simulink library "BLE_Library"  (R2017b)
settings: Solver=VariableStepAuto  StartTime=0.0  StopTime=10.0  RelTol=1e-3
values from neighbouring files (symbols this model uses):
  D = D/ScaleCoefficient    [BLE_PostLoad.m]    (also in new_BLE_model.m = zeros(N_BLE,N_BLE+1))
undefined symbols (not defined in the file or in its folder): ADV_IND_AccA, ADV_IND_id, BT_Hop_Separation, BT_Samples_Per_Symbol, CONNECT_IND_id, CONNECT_IND_length, F3B672D172DF, F506B10B1B3E, Header, LL_DATA_EMPTY_length, LL_DATA_id, magnitude, Payload, Preamble, Slot_Ts, T_IFS
libraries: BLE_Library x56, simulink x39, commutil2 x29, dspindex x17, commdigbbndfm2 x5, dspsigops x2, commrandsrc3 x2, dspstat3 x2, dspsrcs4 x1, dsparch4 x1, commdigbbndcpm2 x1
(part 4 of 5)

== system BLE_Library/Demodulation, De-whitening, CRC check, PDU/De-whitening, CRC check, Data fields/De-whitening/Subsystem ==
  ChIdx : Inport
  Enable : EnablePort  StatesWhenEnabling=reset
  Initial LFSR generation : MATLAB Function  TreatAsAtomicUnit=on
  LFSR : Outport
  wires:
  ChIdx/1 -> Initial LFSR generation/1(ChIdx)
  Initial LFSR generation/1(LFSR) -> LFSR/1

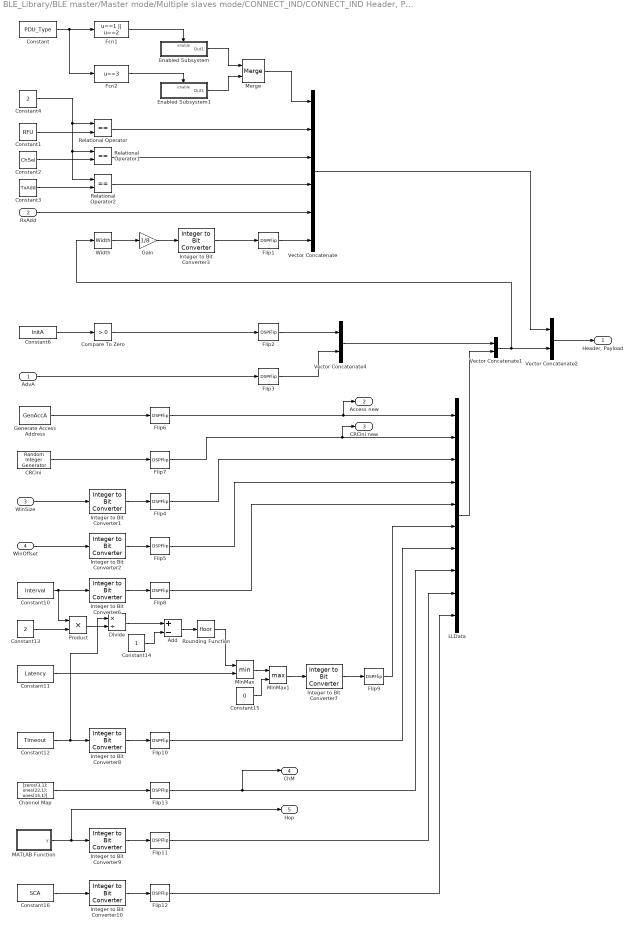
== system BLE_Library/BLE master/Master mode/Multiple slaves mode/CONNECT_IND/CONNECT_IND Header, Payload ==
  AdvA : Inport
  RxAdd : Inport  Port=2
  WinSize : Inport  Port=3
  WinOffset : Inport  Port=4
  Add : Sum  Inputs=+-
  CRCini : commrandsrc3/Random Integer Generator  SetSize=2  SeedSource=Auto  Seed=0  SampleTime=Slot_Ts/24  SamplesPerFrame=24  OutputDataType=boolean  SimulateUsing=Interpreted execution
  Channel Map : Constant  Value=[zeros(3,1); ones(22,1); ones(15,1)]  OutDataTypeStr=boolean  SampleTime=Slot_Ts
  Compare To Zero : simulink/Logic and Bit Operations/Compare To Zero  relop=>  OutDataTypeStr=boolean
  Constant : Constant  Value=PDU_Type  SampleTime=Slot_Ts
  Constant1 : Constant  Value=RFU  SampleTime=Slot_Ts
  Constant10 : Constant  Value=Interval  SampleTime=Slot_Ts
  Constant11 : Constant  Value=Latency  SampleTime=Slot_Ts
  Constant12 : Constant  Value=Timeout  SampleTime=Slot_Ts
  Constant13 : Constant  Value=2  SampleTime=Slot_Ts
  Constant14 : Constant  SampleTime=Slot_Ts
  Constant15 : Constant  Value=0  SampleTime=Slot_Ts
  Constant16 : Constant  Value=SCA  SampleTime=Slot_Ts
  Constant2 : Constant  Value=ChSel  SampleTime=Slot_Ts
  Constant3 : Constant  Value=TxAdd  SampleTime=Slot_Ts
  Constant4 : Constant  Value=2  SampleTime=Slot_Ts
  Constant6 : Constant  Value=InitA  VectorParams1D=off  OutDataTypeStr=double  SampleTime=Slot_Ts
  Divide : Product  Inputs=*/
  Enabled Subsystem : Subsystem  TreatAsAtomicUnit=on
  Enabled Subsystem1 : Subsystem  TreatAsAtomicUnit=on
  Fcn1 : Fcn  Expr=u==1 || u==2
  Fcn2 : Fcn  Expr=u==3
  Flip{1..13} (13 alike) : DSPFlip
  Gain : Gain  Gain=1/8
  Generate Access Address : M-S-Function  Priority=2  FunctionName=GenAccA  Parameters=Slot_Ts
  Integer to Bit Converter1 : commutil2/Integer to Bit Converter  nbits=8  signedInputValues=Unsigned  bitOrder=MSB first  outDtype=boolean
  Integer to Bit Converter10 : commutil2/Integer to Bit Converter  nbits=3  signedInputValues=Unsigned  bitOrder=MSB first  outDtype=boolean
  Integer to Bit Converter{2,6..8} (4 alike) : commutil2/Integer to Bit Converter  nbits=16  signedInputValues=Unsigned  bitOrder=MSB first  outDtype=boolean
  Integer to Bit Converter3 : commutil2/Integer to Bit Converter  nbits=8  signedInputValues=Unsigned  bitOrder=MSB first  outDtype=boolean
  Integer to Bit Converter9 : commutil2/Integer to Bit Converter  nbits=5  signedInputValues=Unsigned  bitOrder=MSB first  outDtype=boolean
  LLData : Concatenate  NumInputs=10
  MATLAB Function : MATLAB Function  TreatAsAtomicUnit=on
  Merge : Merge
  MinMax : MinMax  Inputs=2
  MinMax1 : MinMax  Function=max  Inputs=2
  Product : Product
  Relational Operator : RelationalOperator  Operator===  OutDataTypeStr=boolean  RndMeth=Simplest
  Relational Operator1 : RelationalOperator  Operator===  OutDataTypeStr=boolean  RndMeth=Simplest
  Relational Operator2 : RelationalOperator  Operator===  OutDataTypeStr=boolean  RndMeth=Simplest
  Rounding Function : Rounding
  Vector Concatenate : Concatenate  NumInputs=6
  Vector Concatenate1 : Concatenate
  Vector Concatenate2 : Concatenate
  Vector Concatenate4 : Concatenate
  Width : Width
  "Header, Payload" : Outport
  Access new : Outport  Port=2
  CRCini new : Outport  Port=3
  ChM : Outport  Port=4
  Hop : Outport  Port=5
  wires:
  WinOffset/1 -> Integer to Bit Converter2/1
  WinSize/1 -> Integer to Bit Converter1/1
  MATLAB Function/1(y) -> Integer to Bit Converter9/1, Hop/1
  Channel Map/1 -> Flip13/1
  Flip13/1 -> LLData/8, ChM/1
  Constant14/1 -> Add/2
  Constant11/1 -> MinMax/2
  Constant6/1 -> Compare To Zero/1
  Integer to Bit Converter2/1 -> Flip5/1
  Flip5/1 -> LLData/4
  Fcn1/1 -> Enabled Subsystem/Enable
  Product/1 -> Divide/2
  Merge/1 -> Vector Concatenate/1
  Vector Concatenate/1 -> Vector Concatenate2/1
  Integer to Bit Converter7/1 -> Flip9/1
  Constant/1 -> Fcn1/1, Fcn2/1
  Flip7/1 -> CRCini new/1, LLData/2
  Vector Concatenate2/1 -> "Header, Payload"/1
  Constant1/1 -> Relational Operator/2
  Gain/1 -> Integer to Bit Converter3/1
  Constant4/1 -> Relational Operator2/1, Relational Operator1/1, Relational Operator/1
  CRCini/1 -> Flip7/1
  Integer to Bit Converter8/1 -> Flip10/1
  Integer to Bit Converter9/1 -> Flip11/1
  Flip6/1 -> Access new/1, LLData/1
  Integer to Bit Converter1/1 -> Flip4/1
  MinMax1/1 -> Integer to Bit Converter7/1
  AdvA/1 -> Flip3/1
  Constant13/1 -> Product/2
  Enabled Subsystem/1(Out1) -> Merge/1
  Integer to Bit Converter10/1 -> Flip12/1
  Constant10/1 -> Product/1, Integer to Bit Converter6/1
  Constant3/1 -> Relational Operator2/2
  Divide/1 -> Add/1
  Flip12/1 -> LLData/10
  MinMax/1 -> MinMax1/1
  Enabled Subsystem1/1(Out1) -> Merge/2
  Integer to Bit Converter6/1 -> Flip8/1
  Flip1/1 -> Vector Concatenate/6
  Fcn2/1 -> Enabled Subsystem1/Enable
  Add/1 -> Rounding Function/1
  Relational Operator/1 -> Vector Concatenate/2
  Width/1 -> Gain/1
  Flip4/1 -> LLData/3
  Vector Concatenate4/1 -> Vector Concatenate1/1
  Constant12/1 -> Divide/1, Integer to Bit Converter8/1
  Flip8/1 -> LLData/5
  Vector Concatenate1/1 -> Width/1, Vector Concatenate2/2
  Relational Operator2/1 -> Vector Concatenate/4
  Flip11/1 -> LLData/9
  Flip9/1 -> LLData/6
  Constant16/1 -> Integer to Bit Converter10/1
  Flip10/1 -> LLData/7
  Constant2/1 -> Relational Operator1/2
  Constant15/1 -> MinMax1/2
  Flip3/1 -> Vector Concatenate4/2
  LLData/1 -> Vector Concatenate1/2
  Flip2/1 -> Vector Concatenate4/1
  Integer to Bit Converter3/1 -> Flip1/1
  Relational Operator1/1 -> Vector Concatenate/3
  RxAdd/1 -> Vector Concatenate/5
  Generate Access Address/1 -> Flip6/1
  Compare To Zero/1 -> Flip2/1
  Rounding Function/1 -> MinMax/1

== system BLE_Library/BLE master/Master mode/Multiple slaves mode/CONNECT_IND/Subsystem4 ==
  AdvAccAdr : Constant  Value=ADV_IND_AccA  VectorParams1D=off  SampleTime=Slot_Ts
  AdvPreamble : Constant  Value=[0 1 0 1 0 1 0 1]'  VectorParams1D=off  OutDataTypeStr=boolean  SampleTime=Slot_Ts  FramePeriod=Slot_Ts
  "Concatenate Adv Preamble, Access address" : Concatenate  Mode=Multidimensional array
  Flip1 : DSPFlip
  Out1 : Outport
  wires:
  Flip1/1 -> "Concatenate Adv Preamble, Access address"/2
  AdvPreamble/1 -> "Concatenate Adv Preamble, Access address"/1
  "Concatenate Adv Preamble, Access address"/1 -> Out1/1
  AdvAccAdr/1 -> Flip1/1

== system BLE_Library/BLE master/Master mode/Multiple slaves mode/Subsystem/If Action Subsystem ==
  Header : Inport
  PDU : Inport  Port=2
  Action Port : ActionPort
  Constant : Constant  OutDataTypeStr=boolean  SampleTime=Slot_Ts
  Multiport Selector : dspindex/Multiport Selector  rowsOrCols=Rows  idxCellArray={1:48}  idxErrMode=Clip Index
  Multiport Selector1 : dspindex/Multiport Selector  rowsOrCols=Rows  idxCellArray={10}  idxErrMode=Clip Index
  TxAdd : Outport
  AdvA : Outport  Port=2
  ADV OK : Outport  Port=3
  wires:
  Constant/1 -> ADV OK/1
  Header/1 -> Multiport Selector1/1
  Multiport Selector1/1 -> TxAdd/1
  PDU/1 -> Multiport Selector/1
  Multiport Selector/1 -> AdvA/1

== system BLE_Library/BLE master/Master mode/Multiple slaves mode/Subsystem/If Action Subsystem1 ==
  Header : Inport
  PDU : Inport  Port=2
  Action Port : ActionPort
  Compare To Constant : simulink/Logic and Bit Operations/Compare To Constant  relop===  const=48  OutDataTypeStr=boolean
  Compare To Constant1 : simulink/Logic and Bit Operations/Compare To Constant  relop===  const=2  OutDataTypeStr=boolean
  Constant1 : Constant  Value=TxAdd  VectorParams1D=off  OutDataTypeStr=double  SampleTime=Slot_Ts
  Constant2 : Constant  Value=InitA  VectorParams1D=off  OutDataTypeStr=double  SampleTime=Slot_Ts
  Logical Operator : Logic  AllPortsSameDT=off  OutDataTypeStr=boolean
  Multiport Selector : dspindex/Multiport Selector  rowsOrCols=Rows  idxCellArray={1:48, 49:96}  idxErrMode=Clip Index
  Multiport Selector2 : dspindex/Multiport Selector  rowsOrCols=Rows  idxCellArray={9, 10}  idxErrMode=Clip Index
  Relational Operator1 : RelationalOperator  Operator===  OutDataTypeStr=boolean  RndMeth=Simplest
  Relational Operator2 : RelationalOperator  Operator===  OutDataTypeStr=boolean  RndMeth=Simplest
  Sum of Elements1 : Sum  Inputs=+
  ADV OK : Outport
  AdvA : Outport  Port=2
  TxAdd : Outport  Port=3
  wires:
  Compare To Constant1/1 -> Relational Operator2/1
  Logical Operator/1 -> ADV OK/1
  Constant2/1 -> Relational Operator1/2
  Constant1/1 -> Compare To Constant1/1
  Multiport Selector2/1 -> Relational Operator2/2  "RxAdd"
  Multiport Selector/1 -> Relational Operator1/1  "TargA"
  Sum of Elements1/1 -> Compare To Constant/1
  Relational Operator2/1 -> Logical Operator/1
  Compare To Constant/1 -> Logical Operator/2
  Relational Operator1/1 -> Sum of Elements1/1
  Multiport Selector2/2 -> TxAdd/1
  Header/1 -> Multiport Selector2/1
  Multiport Selector/2 -> AdvA/1
  PDU/1 -> Multiport Selector/1

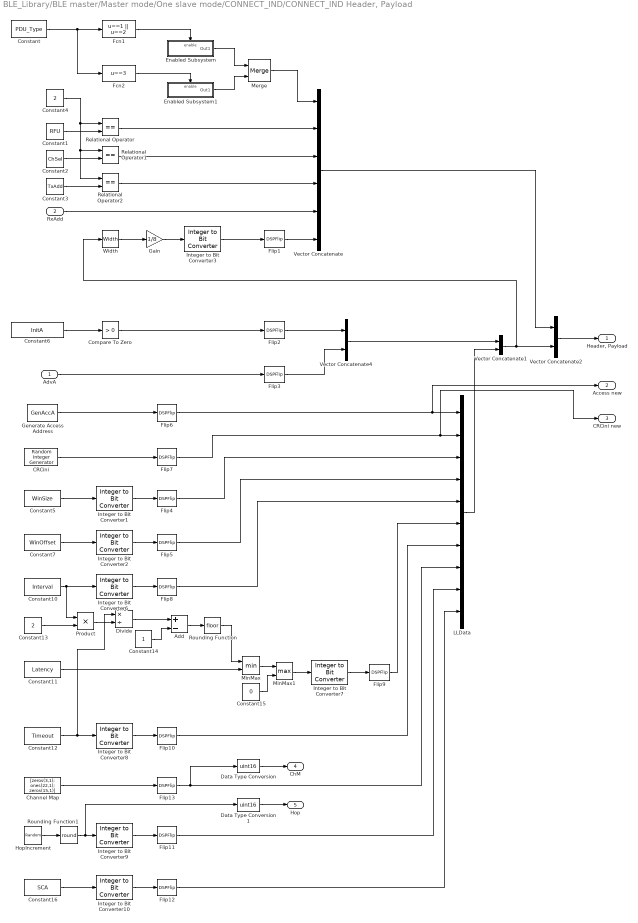
== system BLE_Library/BLE master/Master mode/One slave mode/CONNECT_IND/CONNECT_IND Header, Payload ==
  AdvA : Inport
  RxAdd : Inport  Port=2
  Add : Sum  Inputs=+-
  CRCini : commrandsrc3/Random Integer Generator  SetSize=2  SeedSource=Parameter  Seed=nD  SampleTime=Slot_Ts/24  SamplesPerFrame=24  OutputDataType=boolean  SimulateUsing=Interpreted execution
  Channel Map : Constant  Value=[zeros(3,1); ones(22,1); zeros(15,1)]  OutDataTypeStr=boolean  SampleTime=Slot_Ts
  Compare To Zero : simulink/Logic and Bit Operations/Compare To Zero  relop=>  OutDataTypeStr=boolean
  Constant : Constant  Value=PDU_Type  SampleTime=Slot_Ts
  Constant1 : Constant  Value=RFU  SampleTime=Slot_Ts
  Constant10 : Constant  Value=Interval  SampleTime=Slot_Ts
  Constant11 : Constant  Value=Latency  SampleTime=Slot_Ts
  Constant12 : Constant  Value=Timeout  SampleTime=Slot_Ts
  Constant13 : Constant  Value=2  SampleTime=Slot_Ts
  Constant14 : Constant  SampleTime=Slot_Ts
  Constant15 : Constant  Value=0  SampleTime=Slot_Ts
  Constant16 : Constant  Value=SCA  SampleTime=Slot_Ts
  Constant2 : Constant  Value=ChSel  SampleTime=Slot_Ts
  Constant3 : Constant  Value=TxAdd  SampleTime=Slot_Ts
  Constant4 : Constant  Value=2  SampleTime=Slot_Ts
  Constant5 : Constant  Value=WinSize  SampleTime=Slot_Ts
  Constant6 : Constant  Value=InitA  VectorParams1D=off  OutDataTypeStr=double  SampleTime=Slot_Ts
  Constant7 : Constant  Value=WinOffset  SampleTime=Slot_Ts
  Data Type Conversion : DataTypeConversion  OutDataTypeStr=uint16
  Data Type Conversion1 : DataTypeConversion  OutDataTypeStr=uint16
  Divide : Product  Inputs=*/
  Enabled Subsystem : Subsystem  TreatAsAtomicUnit=on
  Enabled Subsystem1 : Subsystem  TreatAsAtomicUnit=on
  Fcn1 : Fcn  Expr=u==1 || u==2
  Fcn2 : Fcn  Expr=u==3
  Flip{1..13} (13 alike) : DSPFlip
  Gain : Gain  Gain=1/8
  Generate Access Address : M-S-Function  Priority=2  FunctionName=GenAccA  Parameters=Slot_Ts
  HopIncrement : UniformRandomNumber  Minimum=5  Maximum=16  Seed=nD  SampleTime=Slot_Ts
  Integer to Bit Converter1 : commutil2/Integer to Bit Converter  nbits=8  signedInputValues=Unsigned  bitOrder=MSB first  outDtype=boolean
  Integer to Bit Converter10 : commutil2/Integer to Bit Converter  nbits=3  signedInputValues=Unsigned  bitOrder=MSB first  outDtype=boolean
  Integer to Bit Converter{2,6..8} (4 alike) : commutil2/Integer to Bit Converter  nbits=16  signedInputValues=Unsigned  bitOrder=MSB first  outDtype=boolean
  Integer to Bit Converter3 : commutil2/Integer to Bit Converter  nbits=8  signedInputValues=Unsigned  bitOrder=MSB first  outDtype=boolean
  Integer to Bit Converter9 : commutil2/Integer to Bit Converter  nbits=5  signedInputValues=Unsigned  bitOrder=MSB first  outDtype=boolean
  LLData : Concatenate  NumInputs=10
  Merge : Merge
  MinMax : MinMax  Inputs=2
  MinMax1 : MinMax  Function=max  Inputs=2
  Product : Product
  Relational Operator : RelationalOperator  Operator===  OutDataTypeStr=boolean  RndMeth=Simplest
  Relational Operator1 : RelationalOperator  Operator===  OutDataTypeStr=boolean  RndMeth=Simplest
  Relational Operator2 : RelationalOperator  Operator===  OutDataTypeStr=boolean  RndMeth=Simplest
  Rounding Function : Rounding
  Rounding Function1 : Rounding  Operator=round
  Vector Concatenate : Concatenate  NumInputs=6
  Vector Concatenate1 : Concatenate
  Vector Concatenate2 : Concatenate
  Vector Concatenate4 : Concatenate
  Width : Width
  "Header, Payload" : Outport
  Access new : Outport  Port=2
  CRCini new : Outport  Port=3
  ChM : Outport  Port=4
  Hop : Outport  Port=5
  wires:
  Flip13/1 -> LLData/8, Data Type Conversion/1
  Data Type Conversion1/1 -> Hop/1
  Data Type Conversion/1 -> ChM/1
  Constant14/1 -> Add/2
  Constant11/1 -> MinMax/2
  Constant6/1 -> Compare To Zero/1
  Integer to Bit Converter2/1 -> Flip5/1
  Flip5/1 -> LLData/4
  Fcn1/1 -> Enabled Subsystem/Enable
  Product/1 -> Divide/2
  Merge/1 -> Vector Concatenate/1
  Vector Concatenate/1 -> Vector Concatenate2/1
  Integer to Bit Converter7/1 -> Flip9/1
  Constant/1 -> Fcn1/1, Fcn2/1
  Flip7/1 -> LLData/2, CRCini new/1
  HopIncrement/1 -> Rounding Function1/1
  Vector Concatenate2/1 -> "Header, Payload"/1
  Constant1/1 -> Relational Operator/2
  Channel Map/1 -> Flip13/1
  Constant5/1 -> Integer to Bit Converter1/1
  Gain/1 -> Integer to Bit Converter3/1
  Constant4/1 -> Relational Operator2/1, Relational Operator1/1, Relational Operator/1
  Constant7/1 -> Integer to Bit Converter2/1
  CRCini/1 -> Flip7/1
  Integer to Bit Converter8/1 -> Flip10/1
  Integer to Bit Converter9/1 -> Flip11/1
  Flip6/1 -> LLData/1, Access new/1
  Integer to Bit Converter1/1 -> Flip4/1
  MinMax1/1 -> Integer to Bit Converter7/1
  AdvA/1 -> Flip3/1
  Constant13/1 -> Product/2
  Enabled Subsystem/1(Out1) -> Merge/1
  Integer to Bit Converter10/1 -> Flip12/1
  Constant10/1 -> Product/1, Integer to Bit Converter6/1
  Constant3/1 -> Relational Operator2/2
  Divide/1 -> Add/1
  Flip12/1 -> LLData/10
  MinMax/1 -> MinMax1/1
  Enabled Subsystem1/1(Out1) -> Merge/2
  Integer to Bit Converter6/1 -> Flip8/1
  Flip1/1 -> Vector Concatenate/6
  Fcn2/1 -> Enabled Subsystem1/Enable
  Add/1 -> Rounding Function/1
  Relational Operator/1 -> Vector Concatenate/2
  Width/1 -> Gain/1
  Flip4/1 -> LLData/3
  Vector Concatenate4/1 -> Vector Concatenate1/1
  Constant12/1 -> Divide/1, Integer to Bit Converter8/1
  Flip8/1 -> LLData/5
  Vector Concatenate1/1 -> Width/1, Vector Concatenate2/2
  Relational Operator2/1 -> Vector Concatenate/4
  Flip11/1 -> LLData/9
  Flip9/1 -> LLData/6
  Constant16/1 -> Integer to Bit Converter10/1
  Flip10/1 -> LLData/7
  Constant2/1 -> Relational Operator1/2
  Constant15/1 -> MinMax1/2
  Flip3/1 -> Vector Concatenate4/2
  LLData/1 -> Vector Concatenate1/2
  Flip2/1 -> Vector Concatenate4/1
  Integer to Bit Converter3/1 -> Flip1/1
  Rounding Function1/1 -> Integer to Bit Converter9/1, Data Type Conversion1/1
  Relational Operator1/1 -> Vector Concatenate/3
  RxAdd/1 -> Vector Concatenate/5
  Generate Access Address/1 -> Flip6/1
  Compare To Zero/1 -> Flip2/1
  Rounding Function/1 -> MinMax/1

== system BLE_Library/BLE master/Master mode/One slave mode/CONNECT_IND/Subsystem4 ==
  AdvAccAdr : Constant  Value=ADV_IND_AccA  VectorParams1D=off  SampleTime=Slot_Ts
  AdvPreamble : Constant  Value=[0 1 0 1 0 1 0 1]'  VectorParams1D=off  OutDataTypeStr=boolean  SampleTime=Slot_Ts  FramePeriod=Slot_Ts
  "Concatenate Adv Preamble, Access address" : Concatenate  Mode=Multidimensional array
  Flip1 : DSPFlip
  Out1 : Outport
  wires:
  Flip1/1 -> "Concatenate Adv Preamble, Access address"/2
  AdvPreamble/1 -> "Concatenate Adv Preamble, Access address"/1
  "Concatenate Adv Preamble, Access address"/1 -> Out1/1
  AdvAccAdr/1 -> Flip1/1

== system BLE_Library/BLE master/Master mode/One slave mode/Subsystem/If Action Subsystem ==
  Header : Inport
  PDU : Inport  Port=2
  Action Port : ActionPort
  Constant : Constant  OutDataTypeStr=boolean  SampleTime=Slot_Ts
  Multiport Selector : dspindex/Multiport Selector  rowsOrCols=Rows  idxCellArray={1:48}  idxErrMode=Clip Index
  Multiport Selector1 : dspindex/Multiport Selector  rowsOrCols=Rows  idxCellArray={10}  idxErrMode=Clip Index
  TxAdd : Outport
  AdvA : Outport  Port=2
  ADV OK : Outport  Port=3
  wires:
  Constant/1 -> ADV OK/1
  Header/1 -> Multiport Selector1/1
  Multiport Selector1/1 -> TxAdd/1
  PDU/1 -> Multiport Selector/1
  Multiport Selector/1 -> AdvA/1

== system BLE_Library/BLE master/Master mode/One slave mode/Subsystem/If Action Subsystem1 ==
  Header : Inport
  PDU : Inport  Port=2
  Action Port : ActionPort
  Compare To Constant : simulink/Logic and Bit Operations/Compare To Constant  relop===  const=48  OutDataTypeStr=boolean
  Compare To Constant1 : simulink/Logic and Bit Operations/Compare To Constant  relop===  const=2  OutDataTypeStr=boolean
  Constant1 : Constant  Value=TxAdd  VectorParams1D=off  OutDataTypeStr=double  SampleTime=Slot_Ts
  Constant2 : Constant  Value=InitA  VectorParams1D=off  OutDataTypeStr=double  SampleTime=Slot_Ts
  Logical Operator : Logic  AllPortsSameDT=off  OutDataTypeStr=boolean
  Multiport Selector : dspindex/Multiport Selector  rowsOrCols=Rows  idxCellArray={1:48, 49:96}  idxErrMode=Clip Index
  Multiport Selector2 : dspindex/Multiport Selector  rowsOrCols=Rows  idxCellArray={9, 10}  idxErrMode=Clip Index
  Relational Operator1 : RelationalOperator  Operator===  OutDataTypeStr=boolean  RndMeth=Simplest
  Relational Operator2 : RelationalOperator  Operator===  OutDataTypeStr=boolean  RndMeth=Simplest
  Sum of Elements1 : Sum  Inputs=+
  ADV OK : Outport
  AdvA : Outport  Port=2
  TxAdd : Outport  Port=3
  wires:
  Compare To Constant1/1 -> Relational Operator2/1
  Logical Operator/1 -> ADV OK/1
  Constant2/1 -> Relational Operator1/2
  Constant1/1 -> Compare To Constant1/1
  Multiport Selector2/1 -> Relational Operator2/2  "RxAdd"
  Multiport Selector/1 -> Relational Operator1/1  "TargA"
  Sum of Elements1/1 -> Compare To Constant/1
  Relational Operator2/1 -> Logical Operator/1
  Compare To Constant/1 -> Logical Operator/2
  Relational Operator1/1 -> Sum of Elements1/1
  Multiport Selector2/2 -> TxAdd/1
  Header/1 -> Multiport Selector2/1
  Multiport Selector/2 -> AdvA/1
  PDU/1 -> Multiport Selector/1

== system BLE_Library/BLE slave/Battery Status/Subsystem7/Subsystem6/If Action Subsystem2 ==
  In1 : Inport
  In2 : Inport  Port=2
  Action Port : ActionPort
  Constant : Constant  SampleTime=-1
  Divide1 : Product  Inputs=*/
  Sum : Sum  Inputs=|+-
  Out1 : Outport  OutputWhenDisabled=reset  InitialOutput=0
  wires:
  Constant/1 -> Sum/1
  In1/1 -> Sum/2
  Sum/1 -> Divide1/1
  In2/1 -> Divide1/2
  Divide1/1 -> Out1/1

== system BLE_Library/BLE slave/Battery Status/Subsystem7/Subsystem6/If Action Subsystem3 ==
  In1 : Inport
  In2 : Inport  Port=2
  Action Port : ActionPort
  Divide1 : Product  Inputs=*/
  Out1 : Outport  OutputWhenDisabled=reset  InitialOutput=0
  wires:
  In1/1 -> Divide1/1
  In2/1 -> Divide1/2
  Divide1/1 -> Out1/1

== system BLE_Library/BLE master/Master mode/Multiple slaves mode/CONNECT_IND/CONNECT_IND Header, Payload/Enabled Subsystem ==
  Enable : EnablePort
  "CONNECT_IND, AUX_CONNECT_REQ" : Constant  Value=[1 0 1 0]'  OutDataTypeStr=boolean  SampleTime=Slot_Ts
  Out1 : Outport
  wires:
  "CONNECT_IND, AUX_CONNECT_REQ"/1 -> Out1/1

== system BLE_Library/BLE master/Master mode/Multiple slaves mode/CONNECT_IND/CONNECT_IND Header, Payload/Enabled Subsystem1 ==
  Enable : EnablePort
  AUX_CONNECT_RSP : Constant  Value=[0 0 0 1]'  OutDataTypeStr=boolean  SampleTime=Slot_Ts
  Out1 : Outport
  wires:
  AUX_CONNECT_RSP/1 -> Out1/1

== system BLE_Library/BLE master/Master mode/One slave mode/CONNECT_IND/CONNECT_IND Header, Payload/Enabled Subsystem ==
  Enable : EnablePort
  "CONNECT_IND, AUX_CONNECT_REQ" : Constant  Value=[1 0 1 0]'  OutDataTypeStr=boolean  SampleTime=Slot_Ts
  Out1 : Outport
  wires:
  "CONNECT_IND, AUX_CONNECT_REQ"/1 -> Out1/1

== system BLE_Library/BLE master/Master mode/One slave mode/CONNECT_IND/CONNECT_IND Header, Payload/Enabled Subsystem1 ==
  Enable : EnablePort
  AUX_CONNECT_RSP : Constant  Value=[0 0 0 1]'  OutDataTypeStr=boolean  SampleTime=Slot_Ts
  Out1 : Outport
  wires:
  AUX_CONNECT_RSP/1 -> Out1/1

== stateflow chart BLE_Library/BLE master/Master mode/Multiple slaves mode/Initiating state control chart ==
  settings: updateMethod=DISCRETE  sampleTime=Slot_Ts  executeAtInitialization=1
  state Standby
    en: ChIdx=37; TxEn=false; RxEn=false; TxPDU_type=CONNECT_IND_id; RxPDU_type=ADV_IND_id;
    T_LLconnSupervision=InitZ; lastUnmappedChannel=uint16(InitZ); TimeoutBound=6*Interval*1250+InitZ; winOffset=WinOffset+InitZ;
    winSize=WinSize+InitZ; connEventCounter=InitZ; t_anchor=InitZ; ConnEstab=InitZ>0; CStatus=InitZ>0; SN=InitZ>0; NESN=InitZ>0;
    transmitSeqNum=InitZ>0; nextExpectedSeqNum=InitZ>0; MD_SN_NESN_out=repmat(InitZ>0,3,1); RxNewData=InitZ<1; TxNewData=InitZ<1;
    scw=scanWindow; dtt=scanWindow; flagg=true; n_max=Nsl; n_slaves=0; nn=0; n_sl=1; n_ADV=0; branch=0; dt_anchor=0; n_ch=0;
  state InitiatingState
    en: RxEn=true;
    n_ADV=n_ADV-1;
    du,ex: T_LLconnSupervision=T_LLconnSupervision+double(T_LLconnSupervision>0);
  state ADV_Received
    en: RxEn=false;
    du,ex: T_LLconnSupervision=T_LLconnSupervision+double(T_LLconnSupervision>0);
  state SendConnParam
    en: TxEn=true;
    du,ex: T_LLconnSupervision=T_LLconnSupervision+double(T_LLconnSupervision>0);
  state AnchorPointCalculated_Initiate_end1_continue2
    en: disp(GenMsg(['M',nD,': anchor point set for S',r_sl,' at'],(Dclock*1e6+dt_anchor)*1e-3));
    du,ex: T_LLconnSupervision=T_LLconnSupervision+double(T_LLconnSupervision>0);
  state TimeFrame_select
    en: nn=nn+1; tnn1=t_anchor(nn); dt=round(tnn1-Dclock*1e6);
    du,ex: T_LLconnSupervision=T_LLconnSupervision+double(T_LLconnSupervision>0);
  state AnchorPoint_ConnectionEvent_start_Send_start
    en: ChIdx=getChIdx(lastUnmappedChannel(nn),Hop(nn),ChM(:,nn)); lastUnmappedChannel(nn)=ChIdx;
    TxEn=true; tnn2=tnn1+LL_DATA_EMPTY_length; dt=tnn2-Dclock*1e6;
    du,ex: T_LLconnSupervision=T_LLconnSupervision+double(T_LLconnSupervision>0);
  state idx=getChIdx(idx_1,didx,chMap) [function]
    (default) -> (junction 253) : {idx=mod(idx_1+didx,37);}
    (junction 253) -> (junction 257) [order 1] : [chMap(idx+1)==1]
    (junction 253) -> (junction 275) [order 2] : {idxRemap=mod(idx,sum(chMap));
        | ind=-1; k=1;}
    (junction 274) -> (junction 281) [order 1] : [chMap(k)==1]{ind=ind+1;}
    (junction 276) -> (junction 274) [order 1] : [k<41]
    (junction 281) -> (junction 277) [order 2]
    (junction 275) -> (junction 276)
    (junction 274) -> (junction 277) [order 2]
    (junction 281) -> (junction 288) [order 1] : [idxRemap==ind]{idx=uint16(k-1);k=40;}
    (junction 277) -> (junction 276) : {k=k+1;}
    (junction 276) -> (junction 278) [order 2]
    (junction 288) -> (junction 277)
  state Send_end
    en: TxEn=false; tnn3=tnn2+T_IFS; dt=tnn3-Dclock*1e6;
    du,ex: T_LLconnSupervision=T_LLconnSupervision+double(T_LLconnSupervision>0);
  state Receive_start
    en: RxEn=true; tnn4=tnn3+LL_DATA_EMPTY_length; dt=tnn4-Dclock*1e6;
    du,ex: T_LLconnSupervision=T_LLconnSupervision+double(T_LLconnSupervision>0);
  state Receive_continue
    en: dt=tnn4+Length-Dclock*1e6;
    du,ex: T_LLconnSupervision=T_LLconnSupervision+double(T_LLconnSupervision>0);
  (default) -> Standby
  (junction 442) -> Standby
  (junction 488) -> (junction 442)
  Standby -> InitiatingState : [TurnOn]{disp(GenMsg(['M',nD,': initiating state entered at'],Dclock*1e3))}
  InitiatingState -> (junction 187) : [after(scw,tick) || ADVreceived]
  (junction 187) -> (junction 1215) [order 1] : [ADVreceived && RxEn]
      | {n_slaves=n_slaves+1;}
  (junction 1215) -> (junction 1216) [order 2] : {n_sl=nn;}
  (junction 1216) -> ADV_Received
  (junction 187) -> (junction 188) [order 2] : [~ADVreceived]
      | {RxEn=false;}
  (junction 1215) -> (junction 1218) [order 1] : [flagg]
  (junction 1214) -> (junction 1216)
  ADV_Received -> (junction 668) : [after(T_IFS,tick)]{r_sl=GenM(GetSInd(slave_AdvAs, slave_Names, AdvA(:,n_sl))); disp(GenMsg(['M',nD,': advertising packet received from S',r_sl,' at'],Dclock*1e3-T_IFS*1e-3))}
  (junction 437) -> InitiatingState
  (junction 7) -> InitiatingState [order 1] : [ChIdx<39]
      | {ChIdx=ChIdx+1;}
  (junction 1218) -> (junction 1214) : {n_sl=min(n_slaves, n_max);}
  (junction 668) -> (junction 666) [order 2]
  (junction 666) -> (junction 672) [order 2] : {n_slaves=n_slaves-1;}
  (junction 668) -> SendConnParam [order 1] : [n_slaves<2]{dt_anchor=1250*(1+WinOffset)+floor((WinSize*1250+1)*mod(rand(1,1)*nD,1));
      | t_anchor(1)=Dclock*1e6+CONNECT_IND_length+dt_anchor;
      | t_anchor=t_anchor(1)+2500*(cumsum(InitZ+1)-1); n_max=floor(Interval/2);}
  (junction 666) -> (junction 670) [order 1] : [n_slaves<=n_max]
      | {dt_anchor=t_anchor(n_sl)-Dclock*1e6-CONNECT_IND_length;}
  (junction 672) -> (junction 648)
  (junction 7) -> (junction 437) [order 2] : {ChIdx=37;}
  (junction 188) -> (junction 7) [order 2] : after(scanInterval,tick)
  (junction 1171) -> (junction 437) : {ChIdx=37+mod(n_ch,3);}
  (junction 188) -> (junction 947) [order 1] : [n_ADV<1 && n_slaves>0]
  (junction 988) -> SendConnParam : {winOffset(n_sl)=floor(dt_anchor/1250)-1;}
  (junction 670) -> (junction 988) [order 1] : [dt_anchor>0]
  (junction 986) -> (junction 988)
  (junction 670) -> (junction 987) [order 2]
  SendConnParam -> (junction 1001) : [after(CONNECT_IND_length,tick)]{TxEn=false; disp(GenMsg(['M',nD,': connection created with S',r_sl,' at'],Dclock*1e3));
      | T_LLconnSupervision(n_sl)=1; CStatus(n_sl)=true;}
  (junction 987) -> (junction 986) : {dt_anchor=dt_anchor+Interval*1250;}
  (junction 1178) -> (junction 1168)
  (junction 1168) -> (junction 1171)
  (junction 951) -> (junction 947)
  (junction 648) -> (junction 951)
  (junction 1177) -> (junction 1178)
  (junction 1174) -> (junction 1168) [order 1] : [dtt>=128]{scw=dtt;}
  (junction 1167) -> (junction 1171) [order 1] : [dtt>scanWindow]{scw=scanWindow;}
  (junction 947) -> (junction 629) : {flagg=false;
      | TxPDU_type=LL_DATA_id; RxPDU_type=LL_DATA_id;}
  (junction 950) -> (junction 951)
  (junction 1174) -> (junction 1177) [order 2] : {scw=0;}
  (junction 1167) -> (junction 1174) [order 2]
  (junction 617) -> (junction 1167) : {n_ADV=n_adv;
      | disp(GenMsg(['M',nD,': initiating state entered at'],Dclock*1e3))}
  (junction 1001) -> (junction 1000) [order 2] : {lastUnmappedChannel(n_sl)=0;
      | n_adv=0;}
  (junction 1000) -> AnchorPointCalculated_Initiate_end1_continue2
  (junction 1001) -> AnchorPointCalculated_Initiate_end1_continue2 [order 1] : [flagg]{dtt=t_anchor(1)-Dclock*1e6-450-CONNECT_IND_length; n_adv=floor(dtt/scanInterval);}
  AnchorPointCalculated_Initiate_end1_continue2 -> (junction 954)
  (junction 954) -> (junction 950) [order 1] : [n_adv<1 && ~flagg]
  (junction 954) -> (junction 614) [order 2]
  (junction 614) -> (junction 617) : [after(T_IFS,tick)]
  (junction 1253) -> TimeFrame_select
  TimeFrame_select -> (junction 689) : [after(dt,tick) || any(T_LLconnSupervision>TimeoutBound)]
  (junction 933) -> (junction 617)
  (junction 696) -> (junction 771)
  (junction 771) -> (junction 629) : {nn=nn-1;}
  (junction 629) -> (junction 966)
  (junction 966) -> (junction 1253) [order 1] : [nn<n_max]
  (junction 487) -> (junction 696) [order 2] : [innd==nn]
  (junction 764) -> (junction 771) [order 1] : [branch==1]
  (junction 651) -> (junction 629)
  (junction 966) -> (junction 970) [order 2]
  (junction 971) -> (junction 1253) : {nn=0; t_anchor=t_anchor+InitZ+Interval*1250;}
  (junction 970) -> (junction 971)
  (junction 487) -> (junction 488) [order 1] : [~any(CStatus)]
  (junction 690) -> (junction 487) : {innd=GetInd(T_LLconnSupervision>TimeoutBound); t_sl=GenM(GetSInd(slave_AdvAs, slave_Names, AdvA(:,innd)));
      | disp(GenMsg(['M',nD,': connection terminated with S',t_sl,' at'],Dclock*1e3-(T_LLconnSupervision(innd)-TimeoutBound(innd)-1)*1e-3));
      | CStatus(innd)=false; ConnEstab(innd)=false;
      | transmitSeqNum(innd)=false; nextExpectedSeqNum(innd)=false; MD_SN_NESN_out(:,innd)=[false; false; false];
      | RxNewData(innd)=true; TxNewData(innd)=true;
      | connEventCounter(innd)=0; T_LLconnSupervision(innd)=0; n_slaves=n_slaves-1;}
  (junction 689) -> (junction 690) [order 1] : [any(T_LLconnSupervision>TimeoutBound)]{branch=1;}
  (junction 487) -> (junction 739) [order 3]
  (junction 441) -> (junction 690)
  (junction 689) -> (junction 1019) [order 2]
  (junction 1039) -> (junction 1082) [order 2]
  (junction 1019) -> (junction 1039) [order 1] : [~CStatus(nn)]{n_ch=n_ch+1;}
  (junction 1082) -> (junction 1266) : {dtt=t_anchor(1)+Interval*1250-Dclock*1e6-300-CONNECT_IND_length;
      | n_adv=floor(dtt/scanInterval);}
  (junction 1039) -> (junction 1267) [order 1] : [nn<n_max]{dtt=2500-300-CONNECT_IND_length;
      | n_adv=floor(dtt/scanInterval);}
  (junction 1019) -> AnchorPoint_ConnectionEvent_start_Send_start [order 2]
  (junction 1266) -> (junction 933) : {TxPDU_type=CONNECT_IND_id; RxPDU_type=ADV_IND_id;}
  (junction 1267) -> (junction 1266)
  (junction 908) -> AnchorPoint_ConnectionEvent_start_Send_start [order 1] : [dt>0]
  (junction 764) -> (junction 908) [order 2] : [branch==2]{dt=tnn2-Dclock*1e6;}
  (junction 739) -> (junction 764)
  (junction 908) -> (junction 910) [order 2]
  (junction 764) -> (junction 760) [order 3]
  AnchorPoint_ConnectionEvent_start_Send_start -> (junction 373) : [after(dt,tick) || any(T_LLconnSupervision>TimeoutBound)]
  (junction 373) -> (junction 441) [order 1] : [any(T_LLconnSupervision>TimeoutBound)]{branch=2;}
  (junction 478) -> (junction 441)
  (junction 373) -> (junction 1237) [order 2]
  (junction 910) -> (junction 1237)
  (junction 1237) -> Send_end : {connEventCounter(nn)=mod(connEventCounter(nn)+1,65536);}
  (junction 760) -> (junction 906) [order 1] : [branch==3]{dt=tnn3-Dclock*1e6;}
  (junction 906) -> Send_end [order 1] : [dt>0]
  (junction 906) -> (junction 913) [order 2]
  (junction 760) -> (junction 761) [order 2]
  Send_end -> (junction 474) : [after(dt,tick) || any(T_LLconnSupervision>TimeoutBound)]
  (junction 474) -> (junction 478) [order 1] : [any(T_LLconnSupervision>TimeoutBound)]{branch=3;}
  (junction 786) -> (junction 478)
  (junction 474) -> Receive_start [order 2]
  (junction 913) -> Receive_start
  (junction 761) -> (junction 904) [order 1] : [branch==4]{dt=tnn4-Dclock*1e6;}
  (junction 904) -> Receive_start [order 1] : [dt>0]
  (junction 904) -> (junction 916) [order 2]
  (junction 761) -> (junction 788) [order 2]
  Receive_start -> (junction 783) : [after(dt,tick) || any(T_LLconnSupervision>TimeoutBound)]
  (junction 783) -> (junction 786) [order 1] : [any(T_LLconnSupervision>TimeoutBound)]{branch=4;}
  (junction 527) -> (junction 786)
  (junction 783) -> Receive_continue [order 2]
  (junction 916) -> Receive_continue
  (junction 788) -> (junction 792) : {dt=tnn4+Length-Dclock*1e6;}
  (junction 792) -> Receive_continue [order 1] : [dt>0]
  (junction 792) -> (junction 919) [order 2]
  Receive_continue -> (junction 525) : [after(dt,tick) || any(T_LLconnSupervision>TimeoutBound)]
  (junction 525) -> (junction 527) [order 1] : [any(T_LLconnSupervision>TimeoutBound)]{branch=5;}
  (junction 525) -> (junction 1235) [order 2]
  (junction 919) -> (junction 1235)
  (junction 1235) -> (junction 1255) : {RxEn=false; r_sl=GenM(GetSInd(slave_AdvAs, slave_Names, AdvA(:,nn)));
      | SN(nn)=MD_SN_NESN_in(2); NESN(nn)=MD_SN_NESN_in(3);}
  (junction 1255) -> (junction 1257) [order 1] : [~ConnEstab(nn) && P_En]
  (junction 1255) -> (junction 1259) [order 2]
  (junction 1257) -> (junction 1258) : {ConnEstab(nn)=true; T_LLconnSupervision(nn)=1; TimeoutBound(nn)=Timeout*10e3;
      | disp(GenMsg(['M',nD,': connection established with S',r_sl,' at'],Dclock*1e3))}
  (junction 1258) -> (junction 1259)
  (junction 1259) -> (junction 385)
  (junction 385) -> (junction 395) [order 1] : [CRC_OK_LL_DATA]{T_LLconnSupervision(nn)=1;
      | disp(GenMsg(['M',nD,': CRC passed from S',r_sl,' at'],Dclock*1e3))}
  (junction 395) -> (junction 390) [order 1] : [SN(nn)==nextExpectedSeqNum(nn)]{RxNewData(nn)=true;
      | nextExpectedSeqNum(nn)=not(nextExpectedSeqNum(nn));}
  (junction 395) -> (junction 390) [order 2] : {RxNewData(nn)=false;}
  (junction 390) -> (junction 388) [order 2] : {TxNewData(nn)=false;}
  (junction 385) -> (junction 573) [order 2] : {disp(GenMsg(['M',nD,': CRC failed from S',r_sl,' at'],Dclock*1e3))}
  (junction 390) -> (junction 388) [order 1] : [NESN(nn)~=transmitSeqNum(nn)]{TxNewData(nn)=true;
      | transmitSeqNum(nn)=not(transmitSeqNum(nn));}
  (junction 573) -> (junction 651) : %ConnectionEvent(nn)_end
  (junction 388) -> (junction 573) : {MD_SN_NESN_out(3,nn)=nextExpectedSeqNum(nn);
      | MD_SN_NESN_out(2,nn)=transmitSeqNum(nn);}
  data: x function_input; m function_output; SlaveList function_input; sInd function_output; SlaveIdxs function_input; SlaveAdvA function_input; str function_input; msg function_output; t function_input; in function_input; index function_output; idx function_output; idx_1 function_input; didx function_input; chMap function_input; ChIdx output uint16; TxEn output; TxPDU_type output; RxEn output; T_IFS parameter; ADVreceived input; scanInterval parameter; scanWindow parameter; WinOffset parameter; WinSize parameter; CONNECT_IND_id parameter double; LL_DATA_id parameter double; lastUnmappedChannel local uint16; ChM input; Hop input; P_En input; CONNECT_IND_length parameter; LL_DATA_EMPTY_length parameter; Interval parameter; RxPDU_type output; ADV_IND_id parameter; nextExpectedSeqNum local; transmitSeqNum local; MD_SN_NESN_in input boolean; Length input; SN local; NESN local; MD_SN_NESN_out output boolean; TxNewData output; RxNewData output; CRC_OK_LL_DATA input boolean; connEventCounter output; T_LLconnSupervision output [..20]; n_sl output; TimeoutBound local; Timeout parameter; Dclock input; TurnOn input; ConnEstab local; nD parameter; t_anchor local; n_ADV local; n_adv local; dt local; nn output; winOffset output; winSize output; dt_anchor local; CStatus local; ind local; innd local; branch local; tnn2 local; tnn3 local; tnn4 local; n_max local; flagg local; tnn1 local; n_slaves local; dtt local; scw local; AdvA input; r_sl local; slave_AdvAs parameter; slave_Names parameter double; t_sl local; n_ch local uint16; Nsl parameter; InitZ input
  function m = GenM(x):
    | function m = GenM(x)
    | 
    | coder.extrinsic('sprintf')
    | m = sprintf('%d',x);
  function sInd = GetSInd(SlaveList,SlaveIdxs,SlaveAdvA):
    | function sInd = GetSInd(SlaveList,SlaveIdxs,SlaveAdvA)
    | 
    | sInd=0;
    | for k=1:size(SlaveList,2)
    |     if sum(SlaveList(:,k)==SlaveAdvA)==48
    |         sInd=SlaveIdxs(k);
    |         break;
    |     end
    | end
  function msg = GenMsg(str,t):
    | function msg = GenMsg(str,t)
    | 
    | coder.extrinsic('sprintf')
    | msg = sprintf("%s %0.3f ms",str,t);
  function index = GetInd(in):
    | function index = GetInd(in)
    | 
    | index=0;
    | for k=1:length(in)
    |     if in(k)
    |         index=k;
    |         break;
    |     end
    | end

== matlab function BLE_Library/BLE master/Master mode/Multiple slaves mode/LL_DATA_empty/MATLAB Function ==
  settings: updateMethod=DISCRETE  sampleTime=Slot_Ts
  data: AccessAddress input boolean size=[32 1]; Preamble output boolean size=[8 1]
function Preamble = fcn(AccessAddress)

if AccessAddress(1)
    Preamble=[true false true false true false true false]';
else
    Preamble=[false true false true false true false true]';
end

== matlab function BLE_Library/CRC, Whitening, Modulation/CRC calculation/CRC generation ==
  data: bin input; CRC output; LFSR input
function CRC = fcn(bin,LFSR)

CRC=false(24,1);
CRC(1)=xor(bin,LFSR(24));
CRC(2)=xor(LFSR(1),CRC(1));
CRC(3)=LFSR(2);
CRC(4)=xor(LFSR(3),CRC(1));
CRC(5)=xor(LFSR(4),CRC(1));
CRC(6)=LFSR(5);
CRC(7)=xor(LFSR(6),CRC(1));
CRC(8:9)=LFSR(7:8);
CRC(10)=xor(LFSR(9),CRC(1));
CRC(11)=xor(LFSR(10),CRC(1));
CRC(12:24)=LFSR(11:23);

== stateflow chart BLE_Library/BLE master/Master mode/One slave mode/Initiating state control chart ==
  settings: updateMethod=DISCRETE  sampleTime=Slot_Ts  executeAtInitialization=1
  state idx=getChIdx(idx_1,didx,chMap) [function]
    (default) -> (junction 253) : {idx=mod(idx_1+didx,37);}
    (junction 253) -> (junction 257) [order 1] : [chMap(idx+1)==1]
    (junction 253) -> (junction 275) [order 2] : {idxRemap=mod(idx,sum(chMap));
        | ind=-1; k=1;}
    (junction 274) -> (junction 281) [order 1] : [chMap(k)==1]{ind=ind+1;}
    (junction 276) -> (junction 274) [order 1] : [k<41]
    (junction 281) -> (junction 277) [order 2]
    (junction 275) -> (junction 276)
    (junction 274) -> (junction 277) [order 2]
    (junction 281) -> (junction 288) [order 1] : [idxRemap==ind]{idx=uint16(k-1);k=40;}
    (junction 277) -> (junction 276) : {k=k+1;}
    (junction 276) -> (junction 278) [order 2]
    (junction 288) -> (junction 277)
  state Standby
    en: ChIdx=37; TxEn=false; RxEn=false;
    TxPDU_type=CONNECT_IND_id; RxPDU_type=ADV_IND_id;
  state InitiatingState
    en: RxEn=true;
  state ADV_Received
    en: RxEn=false;
  state SendConnParam
    en: TxEn=true;
  state ConnectionCreated_Send_end
    en,du,ex: T_LLconnSupervision=T_LLconnSupervision+1;
  state AnchorPoint_ConnectionEvent_start_Send_start
    en: TxEn=true; n_failedMD=0; m=1;
    ChIdx=getChIdx(lastUnmappedChannel,Hop,ChM); lastUnmappedChannel=ChIdx;
    du,ex: m=m+1; T_LLconnSupervision=T_LLconnSupervision+1;
  state Send_start
    en: TxEn=true;
    du,ex: m=m+1; T_LLconnSupervision=T_LLconnSupervision+1;
  state Send_end
    en: TxEn=false;
    du,ex: m=m+1; T_LLconnSupervision=T_LLconnSupervision+1;
  state Receive_start
    en: RxEn=true;
    du,ex: m=m+1; T_LLconnSupervision=T_LLconnSupervision+1;
  state ConnectionEvent_continue_Send_prepare
    du,ex: m=m+1; T_LLconnSupervision=T_LLconnSupervision+1;
  state Receive_end_ConnectionEvent_end
    du,ex: T_LLconnSupervision=T_LLconnSupervision+1;
  (default) -> Standby
  (junction 442) -> Standby
  (junction 488) -> (junction 442)
  Standby -> InitiatingState : [TurnOn]{disp(GenMsg(['M',nD,': initiating state entered at'],Dclock*1e3))}
  (junction 438) -> InitiatingState
  InitiatingState -> (junction 187) : [after(scanWindow,tick) || ADVreceived]
  (junction 187) -> ADV_Received [order 1] : [ADVreceived && RxEn]
  (junction 437) -> (junction 438)
  (junction 187) -> (junction 188) [order 2] : [~ADVreceived]
      | {RxEn=false;}
  ADV_Received -> SendConnParam : after(T_IFS,tick){r_sl=GenM(GetSInd(slave_AdvAs, slave_Names, AdvA));
      | disp(GenMsg(['M',nD,': advertising packet received from S',r_sl,' at'],Dclock*1e3-T_IFS*1e-3))}
  (junction 7) -> InitiatingState [order 1] : [ChIdx<39]
      | {ChIdx=ChIdx+1;}
  (junction 7) -> (junction 437) [order 2] : {ChIdx=37;}
  (junction 188) -> (junction 7) : after(scanInterval,tick)
  SendConnParam -> ConnectionCreated_Send_end : [after(CONNECT_IND_length,tick)]{TxEn=false; TxPDU_type=LL_DATA_id; RxPDU_type=LL_DATA_id;
      | lastUnmappedChannel=0; disp(GenMsg(['M',nD,': connection created with S',r_sl,' at'],Dclock*1e3));
      | transmitSeqNum=false; nextExpectedSeqNum=false; MD_SN_NESN_out=[false; false; false];
      | RxNewData=true; TxNewData=true; T_LLconnSupervision=0;TimeoutBound=6*Interval*1250; ConnEstab=false;}
  (junction 487) -> (junction 488) : {disp(GenMsg(['M',nD,': connection terminated with S',r_sl,' at'],Dclock*1e3))}
  (junction 441) -> (junction 487)
  ConnectionCreated_Send_end -> AnchorPoint_ConnectionEvent_start_Send_start : [after(1250*(1+WinOffset)+floor((WinSize*1250+1)*mod(rand(1,1)*nD,1)),tick)]
      | {connEventCounter=0; disp(GenMsg(['M',nD,': anchor point set for S',r_sl,' at'],Dclock*1e3))}
  (junction 485) -> AnchorPoint_ConnectionEvent_start_Send_start
  AnchorPoint_ConnectionEvent_start_Send_start -> (junction 556)
  Send_start -> (junction 556)
  (junction 556) -> (junction 373) : [after(LL_DATA_EMPTY_length,tick) || T_LLconnSupervision>=TimeoutBound]
  (junction 549) -> Send_start [order 2]
  (junction 373) -> (junction 441) [order 1] : [T_LLconnSupervision>=TimeoutBound]
  (junction 373) -> Send_end [order 2]
  (junction 478) -> (junction 441)
  Send_end -> (junction 474) : [after(T_IFS,tick) || T_LLconnSupervision>=TimeoutBound]
  (junction 474) -> (junction 478) [order 1] : [T_LLconnSupervision>=TimeoutBound]
  (junction 474) -> Receive_start [order 2]
  (junction 527) -> (junction 478)
  Receive_start -> (junction 525) : [after(LL_DATA_EMPTY_length+Length,tick) || T_LLconnSupervision>=TimeoutBound || m>Interval*1250-1-T_IFS]
  (junction 525) -> (junction 527) [order 1] : [T_LLconnSupervision>=TimeoutBound]
  (junction 482) -> (junction 527)
  (junction 525) -> (junction 632) [order 2] : {RxEn=false;
      | MD=MD_SN_NESN_in(1); SN=MD_SN_NESN_in(2); NESN=MD_SN_NESN_in(3);}
  (junction 632) -> (junction 634) [order 1] : [~ConnEstab && P_En]
  (junction 632) -> (junction 636) [order 2]
  (junction 634) -> (junction 635) : {ConnEstab=true; T_LLconnSupervision=0; TimeoutBound=Timeout*10e3;
      | disp(GenMsg(['M',nD,': connection established with S',r_sl,' at'],Dclock*1e3))}
  (junction 635) -> (junction 636)
  (junction 636) -> (junction 385)
  (junction 385) -> (junction 395) [order 1] : [CRC_OK_LL_DATA]{n_failedMD=0; T_LLconnSupervision=0;
      | disp(GenMsg(['M',nD,': CRC passed from S',r_sl,' at'],Dclock*1e3))}
  (junction 395) -> (junction 390) [order 1] : [SN==nextExpectedSeqNum]{RxNewData=true;
      | nextExpectedSeqNum=not(nextExpectedSeqNum);}
  (junction 395) -> (junction 390) [order 2] : {RxNewData=false;}
  (junction 390) -> (junction 388) [order 2] : {TxNewData=false;}
  (junction 385) -> (junction 678) [order 2] : {n_failedMD=n_failedMD+1;
      | disp(GenMsg(['M',nD,': CRC failed from S',r_sl,' at'],Dclock*1e3))}
  (junction 390) -> (junction 388) [order 1] : [NESN~=transmitSeqNum]{TxNewData=true;
      | transmitSeqNum=not(transmitSeqNum);}
  (junction 678) -> (junction 605) [order 1] : [m>Interval*1250-1-T_IFS]
  (junction 682) -> (junction 678)
  (junction 605) -> Receive_end_ConnectionEvent_end
  (junction 678) -> (junction 647) [order 2]
  (junction 680) -> (junction 682) [order 1] : [m>Interval*1250-1-T_IFS]
  (junction 668) -> (junction 646) [order 1] : [P_En]
  (junction 647) -> (junction 668) [order 2]
  (junction 646) -> (junction 656)
  (junction 668) -> (junction 675) [order 2]
  (junction 647) -> (junction 573) [order 1] : [NDM]
  (junction 656) -> (junction 573) [order 1] : [n_failedMD<2]
  (junction 680) -> (junction 573) [order 2]
  (junction 388) -> (junction 680) : {MD_SN_NESN_out(3)=nextExpectedSeqNum; MD_SN_NESN_out(2)=transmitSeqNum;}
  (junction 656) -> (junction 673) [order 2]
  (junction 573) -> (junction 564)
  (junction 673) -> (junction 675)
  (junction 564) -> ConnectionEvent_continue_Send_prepare [order 1] : [(NDM || MD) && Interval*1250-m+1>=2*(T_IFS+LL_DATA_EMPTY_length) ]
  (junction 675) -> Receive_end_ConnectionEvent_end
  (junction 564) -> Receive_end_ConnectionEvent_end [order 2]
  ConnectionEvent_continue_Send_prepare -> (junction 549) : [after(T_IFS,tick) || T_LLconnSupervision>=TimeoutBound]
  (junction 549) -> (junction 551) [order 1] : [T_LLconnSupervision>=TimeoutBound]
  Receive_end_ConnectionEvent_end -> (junction 434) : [after(Interval*1250-m+1,tick) || T_LLconnSupervision>=TimeoutBound]
  (junction 434) -> (junction 482) [order 1] : [T_LLconnSupervision>=TimeoutBound]
  (junction 551) -> (junction 434)
  (junction 434) -> (junction 481) [order 2] : {connEventCounter=mod(connEventCounter+1,65536);}
  (junction 481) -> (junction 485)
  data: idx function_output; idx_1 function_input; didx function_input; chMap function_input; SlaveList function_input; sInd function_output; SlaveIdxs function_input; SlaveAdvA function_input; str function_input; msg function_output; t function_input; x function_input; k function_output; ChIdx output uint16; TxEn output; TxPDU_type output; RxEn output; T_IFS parameter; ADVreceived input; scanInterval parameter; scanWindow parameter; WinOffset parameter; WinSize parameter; CONNECT_IND_id parameter double; LL_DATA_id parameter double; lastUnmappedChannel local uint16; ChM input; Hop input; P_En input; CONNECT_IND_length parameter; LL_DATA_EMPTY_length parameter; Interval parameter; RxPDU_type output; ADV_IND_id parameter; nextExpectedSeqNum local; transmitSeqNum local; MD_SN_NESN_in input boolean; Length input; MD local; SN local; NESN local; MD_SN_NESN_out output boolean; TxNewData output; RxNewData output; CRC_OK_LL_DATA input boolean; connEventCounter output; T_LLconnSupervision output; TimeoutBound local; Timeout parameter; Dclock input; TurnOn input; ConnEstab local; n_failedMD local; m local; nD parameter; AdvA input; slave_AdvAs parameter; slave_Names parameter; r_sl local; NDM parameter
  function sInd = GetSInd(SlaveList,SlaveIdxs,SlaveAdvA):
    | function sInd = GetSInd(SlaveList,SlaveIdxs,SlaveAdvA)
    | 
    | sInd=0;
    | for k=1:size(SlaveList,2)
    |     if sum(SlaveList(:,k)==SlaveAdvA)==48
    |         sInd=SlaveIdxs(k);
    |         break;
    |     end
    | end
  function msg = GenMsg(str,t):
    | function msg = GenMsg(str,t)
    | 
    | coder.extrinsic('sprintf')
    | msg = sprintf("%s %0.3f ms",str,t);
  function k = GenM(x):
    | function k = GenM(x)
    | 
    | coder.extrinsic('sprintf')
    | k = sprintf('%d',x);

== matlab function BLE_Library/BLE master/Master mode/Multiple slaves mode/CONNECT_IND/CONNECT_IND Header, Payload/MATLAB Function ==
  data: y output
function y = random_number

y=1;
coder.extrinsic('bdroot')
coder.extrinsic('get_param')
y=get_param(bdroot,'SimulationTime')*1e6;
rng(y);

y=randi([5 16],1,1);

== matlab function BLE_Library/CRC, Whitening, Modulation/Whitening/Initial LFSR/Initial LFSR generation ==
  settings: updateMethod=DISCRETE  sampleTime=Slot_Ts
  data: ChIdx input; LFSR output boolean
function LFSR = fcn(ChIdx)

% ChIdx -- channel index for initial LFR value

LFSR=true(7,1);

a=ChIdx; %dec2bin convertion
oki=zeros(1,6);
for k=1:6
    if a~=0
        oki(k)=rem(a,2);
        a=fix(a/2);
    else
        break;
    end
end
a=flip(oki);
LFSR(2:7)=a>0;

== matlab function BLE_Library/CRC, Whitening, Modulation/Whitening/Whitening ==
  settings: updateMethod=DISCRETE  sampleTime=Slot_Ts
  data: bin input; bout output; LFSR input; LFSR_new output
function [bout,LFSR_new] = fcn(bin,LFSR)

bout=true;
bout(1)=xor(bin,LFSR(7));

LFSR_new=false(7,1);
LFSR_new(1)=LFSR(7);
LFSR_new(2)=LFSR(1);
LFSR_new(3)=LFSR(2);
LFSR_new(4)=LFSR(3);
LFSR_new(5)=xor(LFSR(4),LFSR(7));
LFSR_new(6)=LFSR(5);
LFSR_new(7)=LFSR(6);

== matlab function BLE_Library/BLE master/Master mode/One slave mode/LL_DATA_empty/MATLAB Function ==
  settings: updateMethod=DISCRETE  sampleTime=Slot_Ts
  data: AccessAddress input boolean size=[32 1]; Preamble output boolean size=[8 1]
function Preamble = fcn(AccessAddress)

if AccessAddress(1)
    Preamble=[true false true false true false true false]';
else
    Preamble=[false true false true false true false true]';
end
